simulink model "Encoder_Zynq"  (R2018a)
settings: Solver=ode3  StartTime=0.0  StopTime=SimulationsDauer  RelTol=1e-3  EnableMultiTasking=on
values from neighbouring files (symbols this model uses):
  f_ISR = 10000    [Script_Encoder_Zynq.m]
  IncPerTurn = 5000    [Script_Encoder_Zynq.m]
  n_max = 6000    [Script_Encoder_Zynq.m]
  OverSamplingFactor = 6    [Script_Encoder_Zynq.m]
  OverSamplingFactorInverse = 1/OverSamplingFactor    (= 0.166666666667)    [Script_Encoder_Zynq.m]
  Periode = 1/Striche_pro_Sekunde    (= 2.4e-06)    [Script_Encoder_Zynq.m]
  Phase_Delay_A = Periode/8    (= 3e-07)    [Script_Encoder_Zynq.m]
  Phase_Delay_B = -Periode/8    (= -3e-07)    [Script_Encoder_Zynq.m]
  PolePair = 4    [Script_Encoder_Zynq.m]
  T_mech = 2e-08    [Script_Encoder_Zynq.m]
  TestDrehzahl_rpm = 5000    [Script_Encoder_Zynq.m]
undefined symbols (not defined in the file or in its folder): DiscIntNeverNeededParam
libraries: dspswit3 x2, powerlib_meascontrol x2, simulink_extras x1, powerlib x1
(part 1 of 2)
settings Model: Creator=Wendel_ELSYS  LastModifiedBy=Wendel
settings DataIOCC: LimitDataPoints=on  SaveFormat=Array
settings OptimizationCC: BlockReduction=off  ConditionallyExecuteInputs=off  DefaultParameterBehavior=Inlined  LifeSpan=inf
settings DebuggingCC: AlgebraicLoopMsg=error  ParameterOverflowMsg=none  SFUnexpectedBacktrackingDiag=warning  SFNoUnconditionalDefaultTransitionDiag=warning  SFExecutionAtInitializationDiag=none
settings HardwareCC: ProdBitPerPointer=32  ProdBitPerSizeT=32  ProdBitPerPtrDiffT=32  ProdLargestAtomicFloat=None  ProdIntDivRoundTo=Undefined  ProdEndianess=Unspecified  ProdWordSize=32  ProdHWDeviceType=ASIC/FPGA->ASIC/FPGA  ProdEqTarget=off
settings ModelReferenceCC: PropagateSignalLabelsOutOfModel=off
settings CodeAppCC: StateflowObjectComments=on
settings GRTTargetCC: TargetLangStandard=C89/C90 (ANSI)  GeneratePreprocessorConditionals=Disable all
settings ConfigComp: CovMetricSettings=dw  CovHtmlReporting=on  CovSaveCumulativeToWorkspaceVar=on  CovSaveSingleToWorkspaceVar=on  CovExternalEMLEnable=off
settings SimscapeCC: SimscapeNormalizeSystem=off

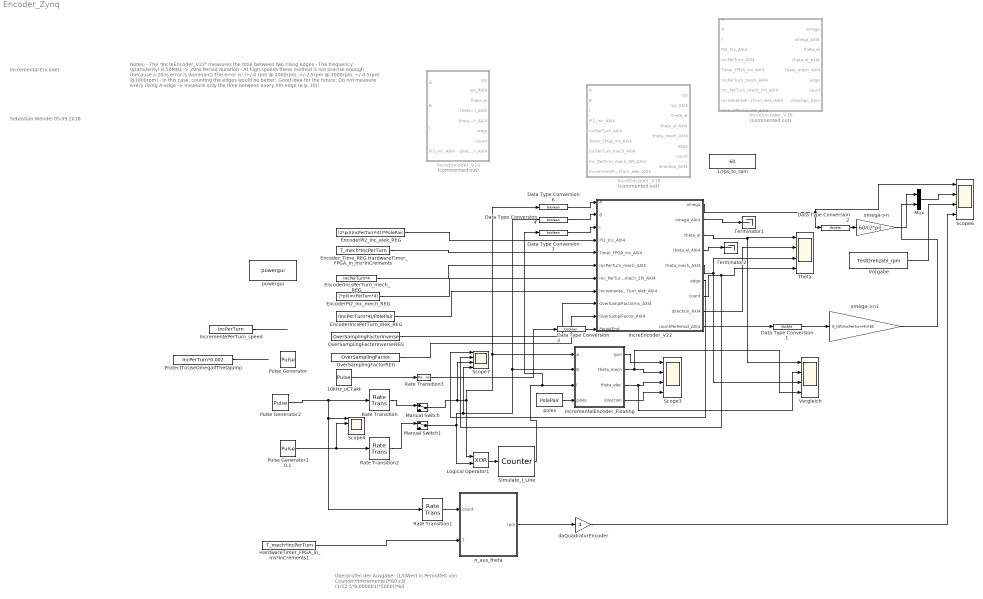
== system Encoder_Zynq ==
  note: Überprüfen der Ausgabe:
      | (1/((Wert in Periodfelt von Counter)*Inkremente))*60
      | z.B. (1/((2.5*0.000001)*5000))*60
  note: Sebastian Wendel
      | 05.09.2018
  note: Notes:
      | - The "IncreEncoder_V22" measures the time between two rising edges
      | - The frequency (granularity) is 50MHz -> 20ns Period duration
      | - At high speeds these method is not precise enough (because a 20ns error is dominant)
      | The error is: (+/-6 rpm @ 5000rpm, +/-2,5rpm @ 3000rpm, +/-0,5rpm @1000rpm)
      | - In this case, counting the edges would be better!
      |
      | Good idea for the future: Do not measure every rising A-edge
      | -> measure only the time between every Xth edge (e.g. 10)!
  note: Incremental Encoder
  1/rps_to_rpm : Constant  Value=60  OutDataTypeStr=double  SampleTime=T_mech
  10kHz_uCTakt : DiscretePulseGenerator  PulseType=Time based  Period=0.000100  PulseWidth=0.0002  SampleTime=T_mech  VectorParams1D=off
  Data Type Conversion1 : DataTypeConversion  OutDataTypeStr=double
  Data Type Conversion2 : DataTypeConversion  OutDataTypeStr=double
  Data Type Conversion{3..4,6..7} (4 alike) : DataTypeConversion  OutDataTypeStr=boolean
  "EncoderIncsPerTurn_elek_REG " : Constant  Value=(IncPerTurn*4)/PolePair  OutDataTypeStr=fixdt(0,16,0)  SampleTime=T_mech
  EncoderIncsPerTurn_mech_REG : Constant  Value=IncPerTurn*4  OutDataTypeStr=fixdt(0,16,0)  SampleTime=T_mech
  EncoderPI2_Inc_elek_REG : Constant  Value=(2*pi/(IncPerTurn*4))*PolePair  OutDataTypeStr=fixdt(0,24,24)  SampleTime=T_mech
  EncoderPI2_Inc_mech_REG : Constant  Value=2*pi/(IncPerTurn*4)  OutDataTypeStr=fixdt(0,24,24)  SampleTime=T_mech
  Encoder_Time_REG HardwareTimer_FPGA_in_ms*InCrements : Constant  Value=T_mech*IncPerTurn  OutDataTypeStr=fixdt(0,32,26)  SampleTime=T_mech
  HardwareTimer_FPGA_in_ms*InCrements1 : Constant  Value=T_mech*IncPerTurn  OutDataTypeStr=double  SampleTime=T_mech
  IncreEncoder_V16 : Subsystem  Commented=on  TreatAsAtomicUnit=on
  IncreEncoder_V18 : Subsystem  Commented=on  TreatAsAtomicUnit=on
  IncreEncoder_V19 : Subsystem  Commented=on  TreatAsAtomicUnit=on
  IncreEncoder_V22 : Subsystem  TreatAsAtomicUnit=on
  IncrementalEncoder_Floating : Subsystem
  IncrementePerTurn_speed : Constant  Value=IncPerTurn  OutDataTypeStr=fixdt(0,16,0)  SampleTime=T_mech
  Logical Operator1 : Logic  Operator=XOR  AllPortsSameDT=off  OutDataTypeStr=boolean
  Manual Switch : ManualSwitch
  Manual Switch1 : ManualSwitch
  Mux : Mux  Inputs=2
  OverSamplingFactorInverseREG : Constant  Value=OverSamplingFactorInverse  OutDataTypeStr=fixdt(0,16,15)  SampleTime=T_mech
  OverSamplingFactorREG : Constant  Value=OverSamplingFactor  OutDataTypeStr=fixdt(0,16,0)  SampleTime=T_mech
  ProtectToUseOmegaIfThetaJump : Constant  Value=IncPerTurn*0.002  OutDataTypeStr=uint16  SampleTime=T_mech
  Pulse Generator : DiscretePulseGenerator  PulseType=Time based  Period=0.01  PulseWidth=50  PhaseDelay=0.00000125  SampleTime=T_mech  VectorParams1D=off
  Pulse Generator1 0.1 : DiscretePulseGenerator  PulseType=Time based  Period=Periode  PulseWidth=50  PhaseDelay=Phase_Delay_B  SampleTime=T_mech  VectorParams1D=off
  Pulse Generator2 : DiscretePulseGenerator  PulseType=Time based  Period=Periode  PulseWidth=50  PhaseDelay=Phase_Delay_A  SampleTime=T_mech  VectorParams1D=off
  Rate Transition{,1..3} (4 alike) : RateTransition  Deterministic=off  OutPortSampleTime=T_mech
  Scope{3..4,6..7} (4 alike) : Scope  NumInputPorts=4
  Simulate_I_Line : dspswit3/Counter  Direction=Up  CountEvent=Either edge  CounterSize=User defined  MaxCount=IncPerTurn*4  InitialCount=0  Output=Hit  HitValue=IncPerTurn*4  ResetInput=off  SamplesPerFrame=1  Ts=1  CntDtype=double  HitDtype=Boolean
  Terminator1 : Terminator
  Terminator2 : Terminator
  Theta : Scope  NumInputPorts=4
  Vergleich : Scope  NumInputPorts=4
  Vorgabe : Constant  Value=TestDrehzahl_rpm
  "daQuadraturEncoder " : Gain  Gain=4
  n_aus_theta : Subsystem  TreatAsAtomicUnit=on
  omega->n : Gain  Gain=60/(2*pi)  OutDataTypeStr=double
  omega->n1 : Gain  Gain=(f_ISR/(IncPerTurn*4))*60  OutDataTypeStr=double
  poles : Constant  Value=PolePair  OutDataTypeStr=uint8  SampleTime=-1
  powergui : powerlib/powergui  Priority=1  SimulationMode=Discrete  SampleTime=T_mech  frequency=60  Iterations=50  frequencyindice=0  Pbase=100e6  ErrMax=1e-4  UnitsV=kV  UnitsW=MW  buscounter=0  FunctionMessages=off  echomessages=off  EnableUseOfTLC=off  CurrentSourceSwitches=off  DisableSnubberDevices=off  DisableRonSwitches=off  DisableVfSwitches=off  DisplayEquations=off  SolverType=Tustin  Interpol=off  ExternalGateDelay=off  methode=off  Ts=0  x0status=blocks  SPID=off  SwTol=0  HookPort=off  RestoreLinks=warning  ResistiveCurrentMeasurement=off  Frange=[0:2:500]  Ylog=off  Xlog=on  ShowGrid=off  save=off  variable=ZData  structure=0  ZoomFFT=on  StartTime=0.0  cycles=1  DisplayStyle=1  fundamental=60  FreqAxis=off  MaxFrequency=1000  frequencyindicesteady=1  RmsSteady=1  display=off
  wires:
  Pulse Generator1 0.1/1 -> Scope4/2, Rate Transition2/1
  Manual Switch1/1 -> Logical Operator1/2, Scope7/4, IncrementalEncoder_Floating/2(B), Data Type Conversion4/1
  Simulate_I_Line/1 -> IncrementalEncoder_Floating/3(I), Data Type Conversion7/1
  Logical Operator1/1 -> Simulate_I_Line/1
  Manual Switch/1 -> Scope7/3, Data Type Conversion6/1, IncrementalEncoder_Floating/1(A), Logical Operator1/1
  Data Type Conversion6/1 -> IncreEncoder_V22/1(A)
  Data Type Conversion4/1 -> IncreEncoder_V22/2(B)
  Data Type Conversion7/1 -> IncreEncoder_V22/3(I)
  IncreEncoder_V22/1(omega) -> Scope6/1, Data Type Conversion2/1
  IncreEncoder_V22/8(direction_AXI4) -> Theta/2
  IncreEncoder_V22/6(edge) -> Scope7/1
  IncreEncoder_V22/7(count) -> Theta/4, Scope7/2
  IncrementalEncoder_Floating/1(rpm) -> Scope3/1
  IncrementalEncoder_Floating/2(theta_mech) -> Vergleich/4, Scope3/2
  IncrementalEncoder_Floating/3(theta_elec) -> Vergleich/2, Scope3/3
  IncrementalEncoder_Floating/4(direction) -> Scope3/4
  poles/1 -> IncrementalEncoder_Floating/4(poles)
  EncoderPI2_Inc_elek_REG/1 -> IncreEncoder_V22/4(PI2_Inc_AXI4)
  IncreEncoder_V22/3(theta_el) -> Theta/1, Vergleich/1
  IncreEncoder_V22/5(theta_mech_AXI4) -> Vergleich/3, Theta/3
  IncreEncoder_V22/4(theta_el_AXI4) -> Terminator2/1
  IncreEncoder_V22/2(omega_AXI4) -> Terminator1/1
  Encoder_Time_REG HardwareTimer_FPGA_in_ms*InCrements/1 -> IncreEncoder_V22/5(Timer_FPGA_ms_AXI4)
  EncoderIncsPerTurn_mech_REG/1 -> IncreEncoder_V22/6(IncPerTurn_mech_AXI4)
  EncoderPI2_Inc_mech_REG/1 -> IncreEncoder_V22/7(Inc_PerTurn_mech_2PI_AXI4)
  IncrementePerTurn_speed/1 -> ?
  "EncoderIncsPerTurn_elek_REG "/1 -> IncreEncoder_V22/8(IncrementePerTurn_elek_AXI4)
  omega->n/1 -> Mux/1
  Data Type Conversion2/1 -> omega->n/1
  HardwareTimer_FPGA_in_ms*InCrements1/1 -> n_aus_theta/2(T)
  Rate Transition1/1 -> n_aus_theta/1(count)
  n_aus_theta/1(rpm) -> "daQuadraturEncoder "/1
  Pulse Generator2/1 -> Rate Transition/1, Scope4/1, Rate Transition1/1
  "daQuadraturEncoder "/1 -> Scope6/4
  ProtectToUseOmegaIfThetaJump/1 -> ?
  Vorgabe/1 -> Scope6/3
  OverSamplingFactorInverseREG/1 -> IncreEncoder_V22/9(OverSamplFactorInv_AXI4)
  OverSamplingFactorREG/1 -> IncreEncoder_V22/10(OverSamplFactor_AXI4)
  Rate Transition2/1 -> Manual Switch1/1
  Rate Transition/1 -> Manual Switch/1
  10kHz_uCTakt/1 -> Rate Transition3/1
  Rate Transition3/1 -> Data Type Conversion3/1
  Data Type Conversion1/1 -> omega->n1/1
  IncreEncoder_V22/9(countPerPeriod_AXI4) -> Data Type Conversion1/1
  Mux/1 -> Scope6/2
  omega->n1/1 -> Mux/2
  Data Type Conversion3/1 -> IncreEncoder_V22/11(PeriodEnd)

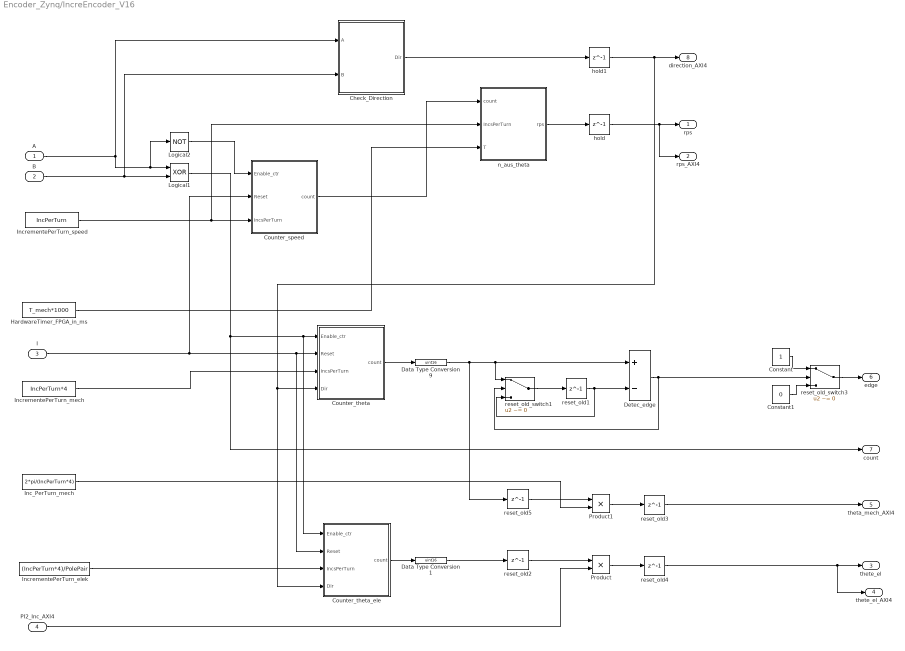
== system Encoder_Zynq/IncreEncoder_V16 ==
  A : Inport
  B : Inport  Port=2
  I : Inport  Port=3
  PI2_Inc_AXI4 : Inport  Port=4
  Check_Direction : Subsystem  TreatAsAtomicUnit=on
  Constant : Constant  OutDataTypeStr=boolean  SampleTime=-1
  Constant1 : Constant  Value=0  OutDataTypeStr=boolean  SampleTime=-1
  Counter_speed : Subsystem  TreatAsAtomicUnit=on
  Counter_theta : Subsystem  TreatAsAtomicUnit=on
  Counter_theta_ele : Subsystem  TreatAsAtomicUnit=on
  Data Type Conversion1 : DataTypeConversion  OutDataTypeStr=uint16
  Data Type Conversion9 : DataTypeConversion  OutDataTypeStr=uint16
  Detec_edge : Sum  Inputs=+-  AccumDataTypeStr=uint8  OutDataTypeStr=uint8
  HardwareTimer_FPGA_in_ms : Constant  Value=T_mech*1000  OutDataTypeStr=fixdt(0,30,24)  SampleTime=T_mech
  Inc_PerTurn_mech : Constant  Value=2*pi/(IncPerTurn*4)  OutDataTypeStr=fixdt(0,24,24)  SampleTime=T_mech
  IncrementePerTurn_elek : Constant  Value=(IncPerTurn*4)/PolePair  OutDataTypeStr=fixdt(0,16,0)  SampleTime=T_mech
  IncrementePerTurn_mech : Constant  Value=IncPerTurn*4  OutDataTypeStr=fixdt(0,16,0)  SampleTime=T_mech
  IncrementePerTurn_speed : Constant  Value=IncPerTurn  OutDataTypeStr=fixdt(0,16,0)  SampleTime=T_mech
  Logical1 : Logic  Operator=XOR  AllPortsSameDT=off  OutDataTypeStr=boolean
  Logical2 : Logic  Operator=NOT  AllPortsSameDT=off  OutDataTypeStr=boolean
  Product : Product  OutDataTypeStr=fixdt(0,24,20)
  Product1 : Product  OutDataTypeStr=fixdt(0,24,20)
  hold : Delay  DelayLength=1
  hold1 : Delay  DelayLength=1
  n_aus_theta : Subsystem  TreatAsAtomicUnit=on
  reset_old{1..5} (5 alike) : Delay  DelayLength=1
  reset_old_switch1 : Switch  Criteria=u2 ~= 0
  reset_old_switch3 : Switch  Criteria=u2 ~= 0
  rps : Outport
  rps_AXI4 : Outport  Port=2
  thete_el : Outport  Port=3
  thete_el_AXI4 : Outport  Port=4
  theta_mech_AXI4 : Outport  Port=5
  edge : Outport  Port=6
  count : Outport  Port=7
  direction_AXI4 : Outport  Port=8
  wires:
  A/1 -> Check_Direction/1(A), Logical2/1, Logical1/1
  B/1 -> Check_Direction/2(B), Logical1/2
  I/1 -> Counter_speed/2(Reset), Counter_theta_ele/2(Reset), Counter_theta/2(Reset)
  IncrementePerTurn_speed/1 -> Counter_speed/3(IncsPerTurn), n_aus_theta/2(IncsPerTurn)
  Check_Direction/1(Dir) -> hold1/1
  hold/1 -> rps_AXI4/1, rps/1
  hold1/1 -> Counter_theta_ele/4(Dir), Counter_theta/4(Dir), direction_AXI4/1
  Counter_theta/1(count) -> Data Type Conversion9/1
  reset_old_switch1/1 -> reset_old1/1
  reset_old1/1 -> reset_old_switch1/3, Detec_edge/2
  reset_old3/1 -> theta_mech_AXI4/1
  Product1/1 -> reset_old3/1
  Inc_PerTurn_mech/1 -> Product1/2
  Product/1 -> reset_old4/1
  Constant/1 -> reset_old_switch3/1
  reset_old_switch3/1 -> edge/1
  Constant1/1 -> reset_old_switch3/3
  Detec_edge/1 -> reset_old_switch3/2, reset_old_switch1/2
  Logical1/1 -> count/1, Counter_theta_ele/1(Enable_ctr), Counter_theta/1(Enable_ctr)
  Counter_speed/1(count) -> n_aus_theta/1(count)
  IncrementePerTurn_mech/1 -> Counter_theta/3(IncsPerTurn)
  n_aus_theta/1(rps) -> hold/1
  Data Type Conversion9/1 -> reset_old5/1, Detec_edge/1, reset_old_switch1/1
  IncrementePerTurn_elek/1 -> Counter_theta_ele/3(IncsPerTurn)
  PI2_Inc_AXI4/1 -> Product/2
  Counter_theta_ele/1(count) -> Data Type Conversion1/1
  reset_old4/1 -> thete_el_AXI4/1, thete_el/1
  Data Type Conversion1/1 -> reset_old2/1
  reset_old2/1 -> Product/1
  reset_old5/1 -> Product1/1
  Logical2/1 -> Counter_speed/1(Enable_ctr)
  HardwareTimer_FPGA_in_ms/1 -> n_aus_theta/3(T)

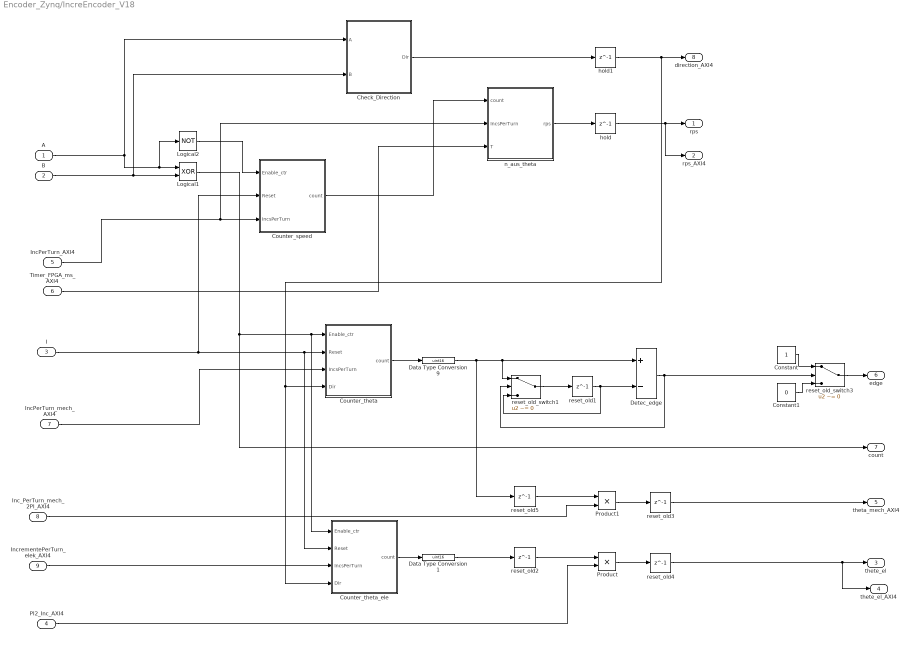
== system Encoder_Zynq/IncreEncoder_V18 ==
  A : Inport
  B : Inport  Port=2
  I : Inport  Port=3
  PI2_Inc_AXI4 : Inport  Port=4
  IncPerTurn_AXI4 : Inport  Port=5
  Timer_FPGA_ms_AXI4 : Inport  Port=6
  IncPerTurn_mech_AXI4 : Inport  Port=7
  Inc_PerTurn_mech_2PI_AXI4 : Inport  Port=8
  IncrementePerTurn_elek_AXI4 : Inport  Port=9
  Check_Direction : Subsystem  TreatAsAtomicUnit=on
  Constant : Constant  OutDataTypeStr=boolean  SampleTime=-1
  Constant1 : Constant  Value=0  OutDataTypeStr=boolean  SampleTime=-1
  Counter_speed : Subsystem  TreatAsAtomicUnit=on
  Counter_theta : Subsystem  TreatAsAtomicUnit=on
  Counter_theta_ele : Subsystem  TreatAsAtomicUnit=on
  Data Type Conversion1 : DataTypeConversion  OutDataTypeStr=uint16
  Data Type Conversion9 : DataTypeConversion  OutDataTypeStr=uint16
  Detec_edge : Sum  Inputs=+-  AccumDataTypeStr=uint8  OutDataTypeStr=uint8
  Logical1 : Logic  Operator=XOR  AllPortsSameDT=off  OutDataTypeStr=boolean
  Logical2 : Logic  Operator=NOT  AllPortsSameDT=off  OutDataTypeStr=boolean
  Product : Product  OutDataTypeStr=fixdt(1,24,20)
  Product1 : Product  OutDataTypeStr=fixdt(1,24,20)
  hold : Delay  DelayLength=1
  hold1 : Delay  DelayLength=1
  n_aus_theta : Subsystem  TreatAsAtomicUnit=on
  reset_old{1..5} (5 alike) : Delay  DelayLength=1
  reset_old_switch1 : Switch  Criteria=u2 ~= 0
  reset_old_switch3 : Switch  Criteria=u2 ~= 0
  rps : Outport
  rps_AXI4 : Outport  Port=2
  thete_el : Outport  Port=3
  thete_el_AXI4 : Outport  Port=4
  theta_mech_AXI4 : Outport  Port=5
  edge : Outport  Port=6
  count : Outport  Port=7
  direction_AXI4 : Outport  Port=8
  wires:
  A/1 -> Check_Direction/1(A), Logical2/1, Logical1/1
  B/1 -> Check_Direction/2(B), Logical1/2
  I/1 -> Counter_speed/2(Reset), Counter_theta_ele/2(Reset), Counter_theta/2(Reset)
  IncPerTurn_AXI4/1 -> Counter_speed/3(IncsPerTurn), n_aus_theta/2(IncsPerTurn)
  Check_Direction/1(Dir) -> hold1/1
  hold/1 -> rps_AXI4/1, rps/1
  hold1/1 -> Counter_theta_ele/4(Dir), Counter_theta/4(Dir), direction_AXI4/1
  Counter_theta/1(count) -> Data Type Conversion9/1
  reset_old_switch1/1 -> reset_old1/1
  reset_old1/1 -> reset_old_switch1/3, Detec_edge/2
  reset_old3/1 -> theta_mech_AXI4/1
  Product1/1 -> reset_old3/1
  Inc_PerTurn_mech_2PI_AXI4/1 -> Product1/2
  Product/1 -> reset_old4/1
  Constant/1 -> reset_old_switch3/1
  reset_old_switch3/1 -> edge/1
  Constant1/1 -> reset_old_switch3/3
  Detec_edge/1 -> reset_old_switch3/2, reset_old_switch1/2
  Logical1/1 -> count/1, Counter_theta_ele/1(Enable_ctr), Counter_theta/1(Enable_ctr)
  Counter_speed/1(count) -> n_aus_theta/1(count)
  IncPerTurn_mech_AXI4/1 -> Counter_theta/3(IncsPerTurn)
  n_aus_theta/1(rps) -> hold/1
  Data Type Conversion9/1 -> reset_old5/1, Detec_edge/1, reset_old_switch1/1
  IncrementePerTurn_elek_AXI4/1 -> Counter_theta_ele/3(IncsPerTurn)
  PI2_Inc_AXI4/1 -> Product/2
  Counter_theta_ele/1(count) -> Data Type Conversion1/1
  reset_old4/1 -> thete_el_AXI4/1, thete_el/1
  Data Type Conversion1/1 -> reset_old2/1
  reset_old2/1 -> Product/1
  reset_old5/1 -> Product1/1
  Logical2/1 -> Counter_speed/1(Enable_ctr)
  Timer_FPGA_ms_AXI4/1 -> n_aus_theta/3(T)

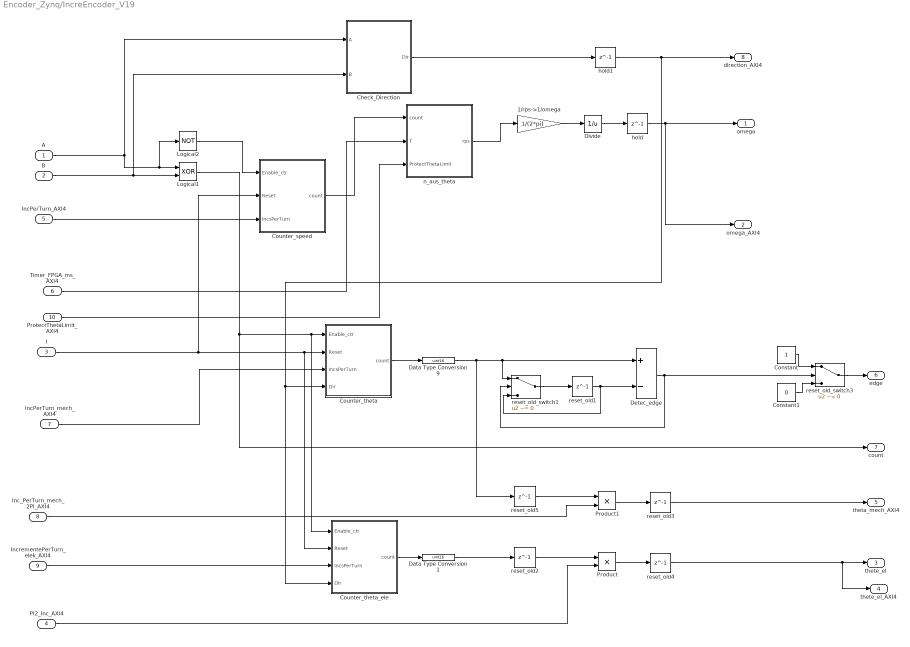
== system Encoder_Zynq/IncreEncoder_V19 ==
  A : Inport
  B : Inport  Port=2
  I : Inport  Port=3
  PI2_Inc_AXI4 : Inport  Port=4
  IncPerTurn_AXI4 : Inport  Port=5
  Timer_FPGA_ms_AXI4 : Inport  Port=6
  IncPerTurn_mech_AXI4 : Inport  Port=7
  Inc_PerTurn_mech_2PI_AXI4 : Inport  Port=8
  IncrementePerTurn_elek_AXI4 : Inport  Port=9
  ProtectThetaLimit_AXI4 : Inport  Port=10
  1/rps->1/omega : Gain  Gain=1/(2*pi)  OutDataTypeStr=fixdt(1,24,18)
  Check_Direction : Subsystem  TreatAsAtomicUnit=on
  Constant : Constant  OutDataTypeStr=boolean  SampleTime=-1
  Constant1 : Constant  Value=0  OutDataTypeStr=boolean  SampleTime=-1
  Counter_speed : Subsystem  TreatAsAtomicUnit=on
  Counter_theta : Subsystem  TreatAsAtomicUnit=on
  Counter_theta_ele : Subsystem  TreatAsAtomicUnit=on
  Data Type Conversion1 : DataTypeConversion  OutDataTypeStr=uint16
  Data Type Conversion9 : DataTypeConversion  OutDataTypeStr=uint16
  Detec_edge : Sum  Inputs=+-  AccumDataTypeStr=uint8  OutDataTypeStr=uint8
  Divide : Math  Operator=reciprocal  OutDataTypeStr=fixdt(1,24,11)  RndMeth=Zero  SaturateOnIntegerOverflow=on
  Logical1 : Logic  Operator=XOR  AllPortsSameDT=off  OutDataTypeStr=boolean
  Logical2 : Logic  Operator=NOT  AllPortsSameDT=off  OutDataTypeStr=boolean
  Product : Product  OutDataTypeStr=fixdt(1,24,20)
  Product1 : Product  OutDataTypeStr=fixdt(1,24,20)
  hold : Delay  DelayLength=1
  hold1 : Delay  DelayLength=1
  n_aus_theta : Subsystem  TreatAsAtomicUnit=on
  reset_old{1..5} (5 alike) : Delay  DelayLength=1
  reset_old_switch1 : Switch  Criteria=u2 ~= 0
  reset_old_switch3 : Switch  Criteria=u2 ~= 0
  omega : Outport
  omega_AXI4 : Outport  Port=2
  thete_el : Outport  Port=3
  thete_el_AXI4 : Outport  Port=4
  theta_mech_AXI4 : Outport  Port=5
  edge : Outport  Port=6
  count : Outport  Port=7
  direction_AXI4 : Outport  Port=8
  wires:
  A/1 -> Check_Direction/1(A), Logical2/1, Logical1/1
  B/1 -> Check_Direction/2(B), Logical1/2
  I/1 -> Counter_speed/2(Reset), Counter_theta_ele/2(Reset), Counter_theta/2(Reset)
  IncPerTurn_AXI4/1 -> Counter_speed/3(IncsPerTurn)
  Check_Direction/1(Dir) -> hold1/1
  hold/1 -> omega_AXI4/1, omega/1
  hold1/1 -> Counter_theta_ele/4(Dir), Counter_theta/4(Dir), direction_AXI4/1
  Counter_theta/1(count) -> Data Type Conversion9/1
  reset_old_switch1/1 -> reset_old1/1
  reset_old1/1 -> reset_old_switch1/3, Detec_edge/2
  reset_old3/1 -> theta_mech_AXI4/1
  Product1/1 -> reset_old3/1
  Inc_PerTurn_mech_2PI_AXI4/1 -> Product1/2
  Product/1 -> reset_old4/1
  Constant/1 -> reset_old_switch3/1
  reset_old_switch3/1 -> edge/1
  Constant1/1 -> reset_old_switch3/3
  Detec_edge/1 -> reset_old_switch3/2, reset_old_switch1/2
  Logical1/1 -> count/1, Counter_theta_ele/1(Enable_ctr), Counter_theta/1(Enable_ctr)
  Counter_speed/1(count) -> n_aus_theta/1(count)
  IncPerTurn_mech_AXI4/1 -> Counter_theta/3(IncsPerTurn)
  n_aus_theta/1(rps) -> 1/rps->1/omega/1
  Data Type Conversion9/1 -> reset_old5/1, Detec_edge/1, reset_old_switch1/1
  IncrementePerTurn_elek_AXI4/1 -> Counter_theta_ele/3(IncsPerTurn)
  PI2_Inc_AXI4/1 -> Product/2
  Counter_theta_ele/1(count) -> Data Type Conversion1/1
  reset_old4/1 -> thete_el_AXI4/1, thete_el/1
  Data Type Conversion1/1 -> reset_old2/1
  reset_old2/1 -> Product/1
  reset_old5/1 -> Product1/1
  Logical2/1 -> Counter_speed/1(Enable_ctr)
  Timer_FPGA_ms_AXI4/1 -> n_aus_theta/2(T)
  Divide/1 -> hold/1
  1/rps->1/omega/1 -> Divide/1
  ProtectThetaLimit_AXI4/1 -> n_aus_theta/3(ProtectThetaLimit)

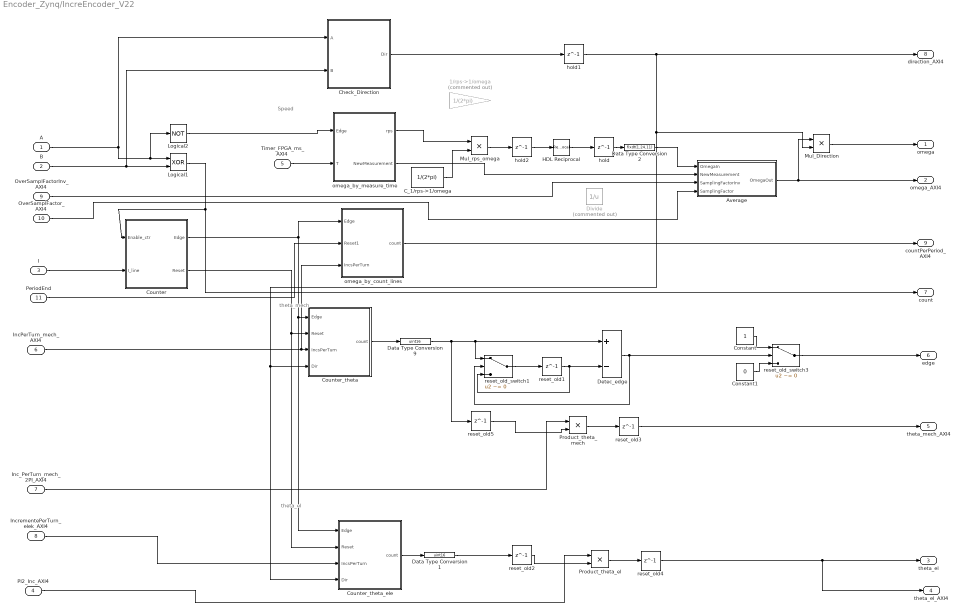
== system Encoder_Zynq/IncreEncoder_V22 ==
  note: Speed
  note: theta_mech
  note: theta_el
  A : Inport
  B : Inport  Port=2
  I : Inport  Port=3
  PI2_Inc_AXI4 : Inport  Port=4
  Timer_FPGA_ms_AXI4 : Inport  Port=5
  IncPerTurn_mech_AXI4 : Inport  Port=6
  Inc_PerTurn_mech_2PI_AXI4 : Inport  Port=7
  IncrementePerTurn_elek_AXI4 : Inport  Port=8
  OverSamplFactorInv_AXI4 : Inport  Port=9
  OverSamplFactor_AXI4 : Inport  Port=10
  PeriodEnd : Inport  Port=11
  1/rps->1/omega : Gain  Commented=on  Gain=1/(2*pi)  OutDataTypeStr=fixdt(1,24,18)
  Average : Subsystem
  C_1/rps->1/omega : Constant  Value=1/(2*pi)  OutDataTypeStr=fixdt(0,16,15)  SampleTime=-1
  Check_Direction : Subsystem  TreatAsAtomicUnit=on
  Constant : Constant  OutDataTypeStr=boolean  SampleTime=-1
  Constant1 : Constant  Value=0  OutDataTypeStr=boolean  SampleTime=-1
  Counter : Subsystem  TreatAsAtomicUnit=on
  Counter_theta : Subsystem  TreatAsAtomicUnit=on
  Counter_theta_ele : Subsystem  TreatAsAtomicUnit=on
  Data Type Conversion1 : DataTypeConversion  OutDataTypeStr=uint16
  Data Type Conversion2 : DataTypeConversion  OutDataTypeStr=fixdt(1,24,11)
  Data Type Conversion9 : DataTypeConversion  OutDataTypeStr=uint16
  Detec_edge : Sum  Inputs=+-  AccumDataTypeStr=uint8  OutDataTypeStr=uint8
  Divide : Math  Commented=on  Operator=reciprocal  OutDataTypeStr=fixdt(1,24,11)  RndMeth=Zero  SaturateOnIntegerOverflow=on
  HDL Reciprocal : Reciprocal
  Logical1 : Logic  Operator=XOR  AllPortsSameDT=off  OutDataTypeStr=boolean
  Logical2 : Logic  Operator=NOT  AllPortsSameDT=off  OutDataTypeStr=boolean
  Mul_Direction : Product  Inputs=**  SaturateOnIntegerOverflow=on  RndMeth=Zero  OutDataTypeStr=Inherit: Same as first input
  Mul_rps_omega : Product  Inputs=**  SaturateOnIntegerOverflow=on  RndMeth=Zero  OutDataTypeStr=Inherit: Same as first input
  Product_theta_el : Product  OutDataTypeStr=fixdt(1,24,20)
  Product_theta_mech : Product  OutDataTypeStr=fixdt(1,24,20)
  hold : Delay  DelayLength=1
  hold1 : Delay  DelayLength=1
  hold2 : Delay  DelayLength=1
  omega_by_count_lines : Subsystem  TreatAsAtomicUnit=on
  omega_by_measure_time : Subsystem  TreatAsAtomicUnit=on
  reset_old{1..5} (5 alike) : Delay  DelayLength=1
  reset_old_switch1 : Switch  Criteria=u2 ~= 0
  reset_old_switch3 : Switch  Criteria=u2 ~= 0
  omega : Outport
  omega_AXI4 : Outport  Port=2
  theta_el : Outport  Port=3
  theta_el_AXI4 : Outport  Port=4
  theta_mech_AXI4 : Outport  Port=5
  edge : Outport  Port=6
  count : Outport  Port=7
  direction_AXI4 : Outport  Port=8
  countPerPeriod_AXI4 : Outport  Port=9
  wires:
  A/1 -> Check_Direction/1(A), Logical2/1, Logical1/1
  B/1 -> Check_Direction/2(B), Logical1/2
  I/1 -> Counter/2(I_line)
  hold/1 -> Data Type Conversion2/1
  hold1/1 -> Mul_Direction/2, Counter_theta_ele/4(Dir), Counter_theta/4(Dir), direction_AXI4/1
  Counter_theta/1(count) -> Data Type Conversion9/1
  reset_old_switch1/1 -> reset_old1/1
  reset_old1/1 -> reset_old_switch1/3, Detec_edge/2
  reset_old3/1 -> theta_mech_AXI4/1
  Product_theta_mech/1 -> reset_old3/1
  Inc_PerTurn_mech_2PI_AXI4/1 -> Product_theta_mech/1
  Product_theta_el/1 -> reset_old4/1
  Constant/1 -> reset_old_switch3/1
  reset_old_switch3/1 -> edge/1
  Constant1/1 -> reset_old_switch3/3
  Detec_edge/1 -> reset_old_switch3/2, reset_old_switch1/2
  Logical1/1 -> count/1, Counter/1(Enable_ctr)
  IncPerTurn_mech_AXI4/1 -> omega_by_count_lines/3(IncsPerTurn), Counter_theta/3(IncsPerTurn)
  omega_by_measure_time/1(rps) -> Mul_rps_omega/1
  Data Type Conversion9/1 -> reset_old5/1, Detec_edge/1, reset_old_switch1/1
  IncrementePerTurn_elek_AXI4/1 -> Counter_theta_ele/3(IncsPerTurn)
  PI2_Inc_AXI4/1 -> Product_theta_el/1
  Counter_theta_ele/1(count) -> Data Type Conversion1/1
  reset_old4/1 -> theta_el_AXI4/1, theta_el/1
  Data Type Conversion1/1 -> reset_old2/1
  reset_old2/1 -> Product_theta_el/2
  reset_old5/1 -> Product_theta_mech/2
  Logical2/1 -> omega_by_measure_time/1(Edge)
  Timer_FPGA_ms_AXI4/1 -> omega_by_measure_time/2(T)
  HDL Reciprocal/1 -> hold/1
  Mul_rps_omega/1 -> hold2/1
  Mul_Direction/1 -> omega/1
  Counter/2(Reset) -> Counter_theta_ele/2(Reset), Counter_theta/2(Reset)
  Counter/1(Edge) -> omega_by_count_lines/1(Edge), Counter_theta_ele/1(Edge), Counter_theta/1(Edge)
  C_1/rps->1/omega/1 -> Mul_rps_omega/2
  hold2/1 -> HDL Reciprocal/1
  Check_Direction/1(Dir) -> hold1/1
  OverSamplFactorInv_AXI4/1 -> Average/3(SamplingFactorInv)
  omega_by_measure_time/2(NewMeasurement) -> Average/2(NewMeasurement)
  OverSamplFactor_AXI4/1 -> Average/4(SamplingFactor)
  Average/1(OmegaOut) -> omega_AXI4/1, Mul_Direction/1
  Data Type Conversion2/1 -> Average/1("OmegaIn ")
  PeriodEnd/1 -> omega_by_count_lines/2(Reset1)
  omega_by_count_lines/1(count) -> countPerPeriod_AXI4/1

== system Encoder_Zynq/IncrementalEncoder_Floating ==
  A : Inport
  B : Inport  Port=2
  I : Inport  Port=3
  poles : Inport  Port=4
  Add : Sum  Inputs=+-  OutDataTypeStr=fixdt(1,16,0)
  Counter3 : dspswit3/Counter  Direction=Up  CountEvent=Either edge  CounterSize=User defined  MaxCount=IncPerTurn*4  InitialCount=0  Output=Count  HitValue=32  ResetInput=on  SamplesPerFrame=1  Ts=1  CntDtype=double  HitDtype=Logical
  CutTheta_0_2PI : Subsystem
  Edge Detector2 : powerlib_meascontrol/Logic/Edge Detector  model=Rising  ic=0  Ts=-1
      settings: SourceProductName=Simscape Power Systems  SourceProductBaseCode=PS
  Edge Detector3 : powerlib_meascontrol/Logic/Edge Detector  model=Rising  ic=0  Ts=-1
      settings: SourceProductName=Simscape Power Systems  SourceProductBaseCode=PS
  Logical Operator1 : Logic  Operator=XOR  AllPortsSameDT=off  OutDataTypeStr=boolean
  Logical Operator3 : Logic  AllPortsSameDT=off  OutDataTypeStr=boolean
  Logical Operator4 : Logic  Operator=NOT  AllPortsSameDT=off  OutDataTypeStr=boolean
  Logical Operator5 : Logic  AllPortsSameDT=off  OutDataTypeStr=boolean
  Logical Operator6 : Logic  Operator=NOT  AllPortsSameDT=off  OutDataTypeStr=boolean
  Product : Product
  S-R Flip-Flop1 : simulink_extras/Flip Flops/S-R Flip-Flop  initial_condition=0
  Scope1 : Scope  NumInputPorts=4
  cut_theta_2pi : Gain  Gain=(2*pi)/IncPerTurn
  cut_theta_2pi1 : Gain  Gain=(2*pi)/IncPerTurn
  n_aus_theta_v4 : Subsystem
  rpm : Outport
  theta_mech : Outport  Port=2
  theta_elec : Outport  Port=3
  direction : Outport  Port=4
  wires:
  I/1 -> Counter3/2
  Counter3/1 -> cut_theta_2pi/1, Product/1, Scope1/1
  n_aus_theta_v4/1(n) -> rpm/1
  Logical Operator1/1 -> Scope1/4, Counter3/1
  cut_theta_2pi/1 -> Scope1/2, n_aus_theta_v4/1(theta), theta_mech/1
  Product/1 -> cut_theta_2pi1/1
  poles/1 -> Product/2
  cut_theta_2pi1/1 -> CutTheta_0_2PI/1(In1)
  CutTheta_0_2PI/1(Out1) -> theta_elec/1
  Edge Detector2/1 -> Logical Operator3/1
  Logical Operator4/1 -> Logical Operator3/2
  Logical Operator3/1 -> S-R Flip-Flop1/1
  Edge Detector3/1 -> Logical Operator5/1
  Logical Operator6/1 -> Logical Operator5/2
  Logical Operator5/1 -> S-R Flip-Flop1/2
  S-R Flip-Flop1/1 -> Add/1
  S-R Flip-Flop1/2 -> Add/2
  A/1 -> Logical Operator6/1, Edge Detector2/1, Logical Operator1/1
  B/1 -> Edge Detector3/1, Logical Operator4/1, Logical Operator1/2
  Add/1 -> direction/1

== system Encoder_Zynq/n_aus_theta ==
  count : Inport
  T : Inport  Port=2
  1/rps->1/omega : Gain  Gain=1/(2*pi)  OutDataTypeStr=double
  Add : Sum  Inputs=+-
  Add1 : Sum
  Constant : Constant  Value=0  OutDataTypeStr=double  SampleTime=-1
  Constant1 : Constant  Value=0  OutDataTypeStr=double  SampleTime=-1
  Constant2 : Constant  Value=0  OutDataTypeStr=double  SampleTime=-1
  Divide1 : Product  Inputs=/
  ProtectOverflow_T_count : Switch  Threshold=50
  ProtectOverflow_rps : Switch  Threshold=50  OutDataTypeStr=double
  Scope1 : Scope  NumInputPorts=4
  Scope2 : Scope  NumInputPorts=4
  T_count : Delay  DelayLength=1
  T_count_switch : Switch  Criteria=u2 ~= 0
  count_old : Delay  DelayLength=1
  count_old_switch : Switch  Criteria=u2 ~= 0
  speed_old : Delay  DelayLength=1
  speed_old_switch : Switch  Criteria=u2 ~= 0
  rpm : Outport
  wires:
  count_old_switch/1 -> count_old/1
  count_old/1 -> count_old_switch/3, Add/2
  Constant/1 -> T_count_switch/1
  Add/1 -> speed_old_switch/2, count_old_switch/2, Scope1/1, T_count_switch/2
  Constant1/1 -> ProtectOverflow_T_count/1
  ProtectOverflow_rps/1 -> 1/rps->1/omega/1, Scope2/1
  Constant2/1 -> ProtectOverflow_rps/1
  speed_old_switch/1 -> ProtectOverflow_rps/3, Scope2/3, speed_old/1
  speed_old/1 -> speed_old_switch/3
  T/1 -> Scope2/4, Add1/1
  ProtectOverflow_T_count/1 -> T_count/1
  T_count/1 -> Scope1/4, Add1/2
  Add1/1 -> Scope2/2, speed_old_switch/1, T_count_switch/3
  count/1 -> Add/1, count_old_switch/1
  T_count_switch/1 -> ProtectOverflow_rps/2, Scope1/2, ProtectOverflow_T_count/2, ProtectOverflow_T_count/3
  1/rps->1/omega/1 -> Divide1/1
  Divide1/1 -> rpm/1

== system Encoder_Zynq/IncreEncoder_V16/Check_Direction ==
  A : Inport
  B : Inport  Port=2
  Add : Sum  Inputs=+-  AccumDataTypeStr=fixdt(1,4,0)  OutDataTypeStr=fixdt(1,4,0)
  Add1 : Sum  Inputs=+-  AccumDataTypeStr=fixdt(1,4,0)  OutDataTypeStr=fixdt(1,4,0)
  Add2 : Sum  AccumDataTypeStr=fixdt(1,4,0)  OutDataTypeStr=fixdt(1,4,0)
  Change : Sum  AccumDataTypeStr=fixdt(1,4,0)  OutDataTypeStr=fixdt(1,4,0)
  Change1 : Delay  DelayLength=1
  Save_Direction : Switch  Criteria=u2 ~= 0  Threshold=0.1  OutDataTypeStr=Inherit: Inherit via back propagation
  Scope6 : Scope  NumInputPorts=4
  T_count_switch : Switch  Threshold=1  OutDataTypeStr=Inherit: Inherit via back propagation
  TrnLeft : Sum  Inputs=+-  AccumDataTypeStr=fixdt(1,4,0)  OutDataTypeStr=fixdt(1,4,0)
  TrnRight : Sum  Inputs=+-  AccumDataTypeStr=fixdt(1,4,0)  OutDataTypeStr=fixdt(1,4,0)
  TurnLeft : Constant  Value=-1  OutDataTypeStr=fixdt(1,4,0)  SampleTime=-1
  TurnRight : Constant  OutDataTypeStr=fixdt(1,4,0)  SampleTime=-1
  count_old : Delay  DelayLength=1
  count_old1 : Delay  DelayLength=1
  count_old2 : Delay  DelayLength=1
  count_old_switch : Switch  Criteria=u2 ~= 0  OutDataTypeStr=Inherit: Inherit via back propagation
  count_old_switch1 : Switch  Criteria=u2 ~= 0  OutDataTypeStr=Inherit: Inherit via back propagation
  new_value : Delay  DelayLength=1
  nothing : Constant  Value=0  OutDataTypeStr=fixdt(1,4,0)  SampleTime=-1
  nothing1 : Constant  Value=0  OutDataTypeStr=fixdt(1,4,0)  SampleTime=-1
  speed_old_switch : Switch  Threshold=1  OutDataTypeStr=Inherit: Inherit via back propagation
  Dir : Outport
  wires:
  A/1 -> TrnLeft/2, Add/1, count_old_switch/1
  count_old_switch/1 -> count_old/1
  count_old/1 -> count_old_switch/3, Add/2
  TurnRight/1 -> T_count_switch/1
  Add/1 -> TrnRight/1, count_old_switch/2
  T_count_switch/1 -> Change/1, Add2/1
  Save_Direction/1 -> count_old2/1
  B/1 -> TrnRight/2, Add1/1, count_old_switch1/1
  count_old_switch1/1 -> count_old1/1
  count_old1/1 -> count_old_switch1/3, Add1/2
  Add1/1 -> TrnLeft/1, count_old_switch1/2
  TrnRight/1 -> Scope6/1, T_count_switch/2
  new_value/1 -> Save_Direction/1
  TrnLeft/1 -> speed_old_switch/2, Scope6/2
  TurnLeft/1 -> speed_old_switch/1
  nothing/1 -> speed_old_switch/3
  nothing1/1 -> T_count_switch/3
  speed_old_switch/1 -> Change/2, Add2/2
  Add2/1 -> Scope6/4, new_value/1
  Change/1 -> Change1/1
  Change1/1 -> Scope6/3, Save_Direction/2
  count_old2/1 -> Save_Direction/3, Dir/1

== system Encoder_Zynq/IncreEncoder_V16/Counter_speed ==
  note: 1 for one cycle if edge recognized
  note: Check if count is to small
  note: Check if count is to big
  note: Reset
  note: Count
  Enable_ctr : Inport
  Reset : Inport  Port=2
  IncsPerTurn : Inport  Port=3
  Add1 : Sum  AccumDataTypeStr=int16  OutDataTypeStr=uint16
  Constant1 : Constant  Value=0  OutDataTypeStr=uint16  SampleTime=-1
  Constant2 : Constant  OutDataTypeStr=int8  SampleTime=-1
  Constant3 : Constant  Value=0  OutDataTypeStr=int8  SampleTime=-1
  Constant4 : Constant  Value=10  OutDataTypeStr=uint16  SampleTime=-1
  Detec_edge : Sum  Inputs=+-  AccumDataTypeStr=int8  OutDataTypeStr=int8
  Relational Operator : RelationalOperator  OutDataTypeStr=boolean  RndMeth=Nearest
  Reset_flag : Sum  Inputs=+-  AccumDataTypeStr=uint8  OutDataTypeStr=uint8
  Reset_when_overflow : Sum
  Resett_switch1 : Switch  Criteria=u2 ~= 0
  Resett_switch2 : Switch  Criteria=u2 ~= 0
  reset_old{,1..3} (4 alike) : Delay  DelayLength=1
  reset_old_switch : Switch  Criteria=u2 ~= 0
  reset_old_switch1 : Switch  Criteria=u2 ~= 0
  speed_old_switch1 : Switch  Threshold=1
  count : Outport
  wires:
  Reset/1 -> Reset_flag/1, reset_old_switch/1
  reset_old_switch/1 -> reset_old/1
  reset_old/1 -> reset_old_switch/3, Reset_flag/2
  Reset_flag/1 -> reset_old_switch/2, Resett_switch2/2
  Enable_ctr/1 -> Detec_edge/1, reset_old_switch1/1
  reset_old_switch1/1 -> reset_old1/1
  reset_old1/1 -> reset_old_switch1/3, Detec_edge/2
  Detec_edge/1 -> speed_old_switch1/2, reset_old_switch1/2  "1 for one cycle if edge recognized"
  Add1/1 -> Resett_switch2/3
  reset_old2/1 -> Relational Operator/1, Add1/2, count/1
  speed_old_switch1/1 -> Add1/1
  Constant3/1 -> speed_old_switch1/3
  Constant2/1 -> speed_old_switch1/1
  Constant4/1 -> Reset_when_overflow/1
  Reset_when_overflow/1 -> reset_old3/1
  Resett_switch1/1 -> reset_old2/1
  Relational Operator/1 -> Resett_switch1/2
  Constant1/1 -> Resett_switch2/1, Resett_switch1/1
  IncsPerTurn/1 -> Reset_when_overflow/2
  Resett_switch2/1 -> Resett_switch1/3
  reset_old3/1 -> Relational Operator/2

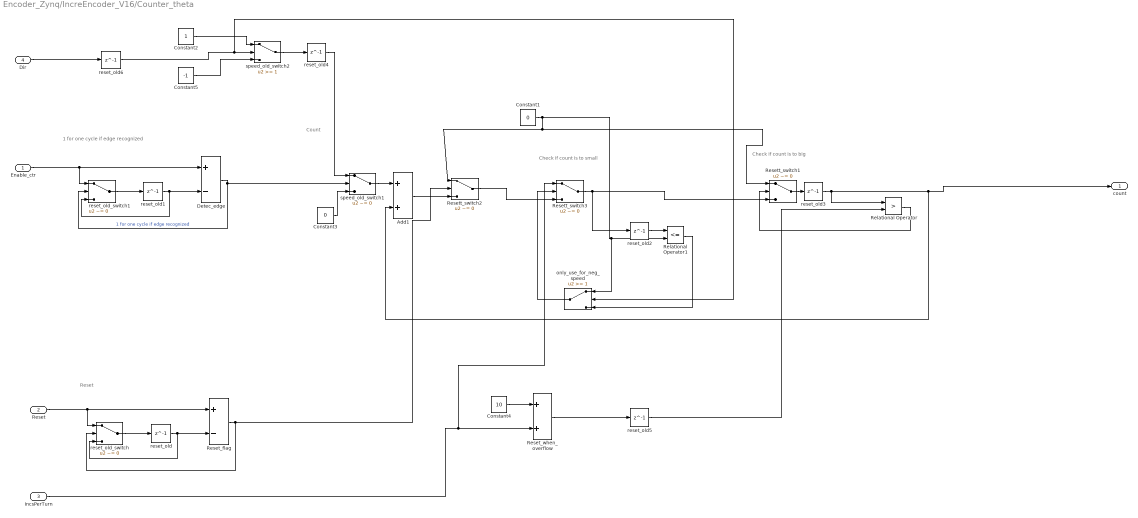
== system Encoder_Zynq/IncreEncoder_V16/Counter_theta ==
  note: 1 for one cycle if edge recognized
  note: Reset
  note: Count
  note: Check if count is to big
  note: Check if count is to small
  Enable_ctr : Inport
  Reset : Inport  Port=2
  IncsPerTurn : Inport  Port=3
  Dir : Inport  Port=4
  Add1 : Sum  AccumDataTypeStr=int16  OutDataTypeStr=int16
  Constant1 : Constant  Value=0  OutDataTypeStr=int16  SampleTime=-1
  Constant2 : Constant  OutDataTypeStr=int16  SampleTime=-1
  Constant3 : Constant  Value=0  OutDataTypeStr=int16  SampleTime=-1
  Constant4 : Constant  Value=10  OutDataTypeStr=int16  SampleTime=-1
  Constant5 : Constant  Value=-1  OutDataTypeStr=int16  SampleTime=-1
  Detec_edge : Sum  Inputs=+-  AccumDataTypeStr=int8  OutDataTypeStr=int8
  Relational Operator : RelationalOperator  Operator=>  OutDataTypeStr=boolean  RndMeth=Nearest
  Relational Operator1 : RelationalOperator  Operator=<=  OutDataTypeStr=boolean  RndMeth=Nearest
  Reset_flag : Sum  Inputs=+-  AccumDataTypeStr=uint8  OutDataTypeStr=uint8
  Reset_when_overflow : Sum  OutDataTypeStr=int16
  Resett_switch1 : Switch  Criteria=u2 ~= 0  OutDataTypeStr=int16
  Resett_switch2 : Switch  Criteria=u2 ~= 0  OutDataTypeStr=int16
  Resett_switch3 : Switch  Criteria=u2 ~= 0  OutDataTypeStr=int16
  only_use_for_neg_speed : Switch  Threshold=1
  reset_old{,1..6} (7 alike) : Delay  DelayLength=1
  reset_old_switch : Switch  Criteria=u2 ~= 0
  reset_old_switch1 : Switch  Criteria=u2 ~= 0
  speed_old_switch1 : Switch  Criteria=u2 ~= 0
  speed_old_switch2 : Switch  Threshold=1
  count : Outport
  wires:
  Reset/1 -> Reset_flag/1, reset_old_switch/1
  reset_old_switch/1 -> reset_old/1
  reset_old/1 -> reset_old_switch/3, Reset_flag/2
  Reset_flag/1 -> reset_old_switch/2, Resett_switch2/2
  Enable_ctr/1 -> Detec_edge/1, reset_old_switch1/1
  reset_old_switch1/1 -> reset_old1/1
  reset_old1/1 -> reset_old_switch1/3, Detec_edge/2
  Detec_edge/1 -> speed_old_switch1/2, reset_old_switch1/2  "1 for one cycle if edge recognized"
  Add1/1 -> Resett_switch2/3
  speed_old_switch1/1 -> Add1/1
  Constant3/1 -> speed_old_switch1/3
  Constant2/1 -> speed_old_switch2/1
  Constant4/1 -> Reset_when_overflow/1
  Reset_when_overflow/1 -> reset_old5/1
  IncsPerTurn/1 -> Resett_switch3/1, Reset_when_overflow/2
  Dir/1 -> reset_old6/1
  Constant5/1 -> speed_old_switch2/3
  speed_old_switch2/1 -> reset_old4/1
  reset_old3/1 -> Add1/2, count/1, Relational Operator/1
  Resett_switch1/1 -> reset_old3/1
  Relational Operator/1 -> Resett_switch1/2
  Constant1/1 -> Resett_switch2/1, Resett_switch1/1, only_use_for_neg_speed/1, Relational Operator1/2
  Resett_switch3/1 -> reset_old2/1, Resett_switch1/3
  Resett_switch2/1 -> Resett_switch3/3
  reset_old2/1 -> Relational Operator1/1
  Relational Operator1/1 -> only_use_for_neg_speed/3
  only_use_for_neg_speed/1 -> Resett_switch3/2
  reset_old4/1 -> speed_old_switch1/1
  reset_old5/1 -> Relational Operator/2
  reset_old6/1 -> only_use_for_neg_speed/2, speed_old_switch2/2

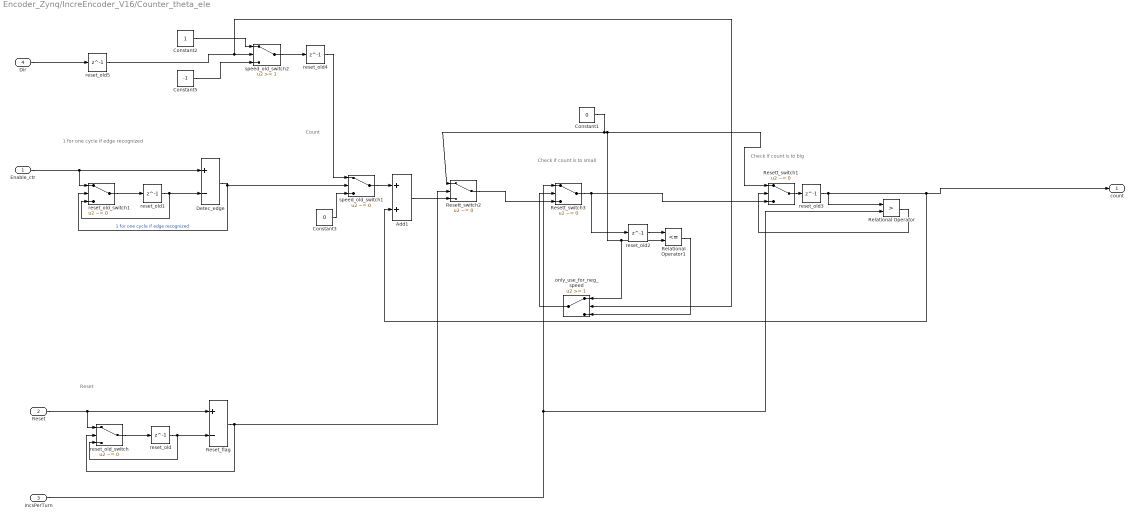
== system Encoder_Zynq/IncreEncoder_V16/Counter_theta_ele ==
  note: 1 for one cycle if edge recognized
  note: Reset
  note: Count
  note: Check if count is to big
  note: Check if count is to small
  Enable_ctr : Inport
  Reset : Inport  Port=2
  IncsPerTurn : Inport  Port=3
  Dir : Inport  Port=4
  Add1 : Sum  AccumDataTypeStr=int16  OutDataTypeStr=int16
  Constant1 : Constant  Value=0  OutDataTypeStr=int16  SampleTime=-1
  Constant2 : Constant  OutDataTypeStr=int16  SampleTime=-1
  Constant3 : Constant  Value=0  OutDataTypeStr=int16  SampleTime=-1
  Constant5 : Constant  Value=-1  OutDataTypeStr=int16  SampleTime=-1
  Detec_edge : Sum  Inputs=+-  AccumDataTypeStr=int8  OutDataTypeStr=int8
  Relational Operator : RelationalOperator  Operator=>  OutDataTypeStr=boolean  RndMeth=Nearest
  Relational Operator1 : RelationalOperator  Operator=<=  OutDataTypeStr=boolean  RndMeth=Nearest
  Reset_flag : Sum  Inputs=+-  AccumDataTypeStr=uint8  OutDataTypeStr=uint8
  Resett_switch1 : Switch  Criteria=u2 ~= 0  OutDataTypeStr=int16
  Resett_switch2 : Switch  Criteria=u2 ~= 0  OutDataTypeStr=int16
  Resett_switch3 : Switch  Criteria=u2 ~= 0  OutDataTypeStr=int16
  only_use_for_neg_speed : Switch  Threshold=1
  reset_old{,1..5} (6 alike) : Delay  DelayLength=1
  reset_old_switch : Switch  Criteria=u2 ~= 0
  reset_old_switch1 : Switch  Criteria=u2 ~= 0
  speed_old_switch1 : Switch  Criteria=u2 ~= 0
  speed_old_switch2 : Switch  Threshold=1
  count : Outport
  wires:
  Reset/1 -> Reset_flag/1, reset_old_switch/1
  reset_old_switch/1 -> reset_old/1
  reset_old/1 -> reset_old_switch/3, Reset_flag/2
  Reset_flag/1 -> reset_old_switch/2, Resett_switch2/2
  Enable_ctr/1 -> Detec_edge/1, reset_old_switch1/1
  reset_old_switch1/1 -> reset_old1/1
  reset_old1/1 -> reset_old_switch1/3, Detec_edge/2
  Detec_edge/1 -> speed_old_switch1/2, reset_old_switch1/2  "1 for one cycle if edge recognized"
  Add1/1 -> Resett_switch2/3
  speed_old_switch1/1 -> Add1/1
  Constant3/1 -> speed_old_switch1/3
  Constant2/1 -> speed_old_switch2/1
  IncsPerTurn/1 -> Resett_switch3/1, Relational Operator/2
  Dir/1 -> reset_old5/1
  Constant5/1 -> speed_old_switch2/3
  speed_old_switch2/1 -> reset_old4/1
  reset_old3/1 -> Add1/2, count/1, Relational Operator/1
  Resett_switch1/1 -> reset_old3/1
  Relational Operator/1 -> Resett_switch1/2
  Constant1/1 -> Resett_switch2/1, only_use_for_neg_speed/1, Relational Operator1/2, Resett_switch1/1
  Resett_switch3/1 -> reset_old2/1, Resett_switch1/3
  Resett_switch2/1 -> Resett_switch3/3
  reset_old2/1 -> Relational Operator1/1
  Relational Operator1/1 -> only_use_for_neg_speed/3
  only_use_for_neg_speed/1 -> Resett_switch3/2
  reset_old4/1 -> speed_old_switch1/1
  reset_old5/1 -> speed_old_switch2/2, only_use_for_neg_speed/2

== system Encoder_Zynq/IncreEncoder_V16/n_aus_theta ==
  count : Inport
  IncsPerTurn : Inport  Port=2
  T : Inport  Port=3
  Add : Sum  Inputs=+-
  Add1 : Sum
  Constant : Constant  Value=0  OutDataTypeStr=fixdt(0,30,24)  SampleTime=-1
  Constant1 : Constant  Value=0  OutDataTypeStr=fixdt(0,30,24)  SampleTime=-1
  Constant2 : Constant  Value=0  OutDataTypeStr=fixdt(0,30,24)  SampleTime=-1
  Gain : Gain  Gain=0.001  ParamDataTypeStr=fixdt(0,16)  OutMin=0  OutMax=0.001*2^16  OutDataTypeStr=fixdt(0,18)
  Product : Product  OutDataTypeStr=Inherit: Same as first input
  ProtectOverflow_T_count : Switch  Threshold=50
  ProtectOverflow_rps : Switch  Threshold=50  OutDataTypeStr=fixdt(0,30,24)
  T_count : Delay  DelayLength=1
  T_count_switch : Switch  Criteria=u2 ~= 0
  count_old : Delay  DelayLength=1
  count_old_switch : Switch  Criteria=u2 ~= 0
  speed_old : Delay  DelayLength=1
  speed_old_switch : Switch  Criteria=u2 ~= 0
  rps : Outport
  wires:
  count_old_switch/1 -> count_old/1
  count_old/1 -> count_old_switch/3, Add/2
  Constant/1 -> T_count_switch/1
  Add/1 -> speed_old_switch/2, count_old_switch/2, T_count_switch/2
  Constant1/1 -> ProtectOverflow_T_count/1
  ProtectOverflow_rps/1 -> rps/1
  Constant2/1 -> ProtectOverflow_rps/1
  speed_old_switch/1 -> ProtectOverflow_rps/3, speed_old/1
  speed_old/1 -> speed_old_switch/3
  IncsPerTurn/1 -> Gain/1
  Gain/1 -> Product/2
  T/1 -> Add1/1
  ProtectOverflow_T_count/1 -> T_count/1
  T_count/1 -> Add1/2
  Product/1 -> speed_old_switch/1
  Add1/1 -> Product/1, T_count_switch/3
  count/1 -> Add/1, count_old_switch/1
  T_count_switch/1 -> ProtectOverflow_rps/2, ProtectOverflow_T_count/2, ProtectOverflow_T_count/3

== system Encoder_Zynq/IncreEncoder_V18/Check_Direction ==
  A : Inport
  B : Inport  Port=2
  Add : Sum  Inputs=+-  AccumDataTypeStr=fixdt(1,4,0)  OutDataTypeStr=fixdt(1,4,0)
  Add1 : Sum  Inputs=+-  AccumDataTypeStr=fixdt(1,4,0)  OutDataTypeStr=fixdt(1,4,0)
  Add2 : Sum  AccumDataTypeStr=fixdt(1,4,0)  OutDataTypeStr=fixdt(1,4,0)
  Change : Sum  AccumDataTypeStr=fixdt(1,4,0)  OutDataTypeStr=fixdt(1,4,0)
  Change1 : Delay  DelayLength=1
  Save_Direction : Switch  Criteria=u2 ~= 0  Threshold=0.1  OutDataTypeStr=Inherit: Inherit via back propagation
  Scope6 : Scope  NumInputPorts=4
  T_count_switch : Switch  Threshold=1  OutDataTypeStr=Inherit: Inherit via back propagation
  TrnLeft : Sum  Inputs=+-  AccumDataTypeStr=fixdt(1,4,0)  OutDataTypeStr=fixdt(1,4,0)
  TrnRight : Sum  Inputs=+-  AccumDataTypeStr=fixdt(1,4,0)  OutDataTypeStr=fixdt(1,4,0)
  TurnLeft : Constant  Value=-1  OutDataTypeStr=fixdt(1,4,0)  SampleTime=-1
  TurnRight : Constant  OutDataTypeStr=fixdt(1,4,0)  SampleTime=-1
  count_old : Delay  DelayLength=1
  count_old1 : Delay  DelayLength=1
  count_old2 : Delay  DelayLength=1
  count_old_switch : Switch  Criteria=u2 ~= 0  OutDataTypeStr=Inherit: Inherit via back propagation
  count_old_switch1 : Switch  Criteria=u2 ~= 0  OutDataTypeStr=Inherit: Inherit via back propagation
  new_value : Delay  DelayLength=1
  nothing : Constant  Value=0  OutDataTypeStr=fixdt(1,4,0)  SampleTime=-1
  nothing1 : Constant  Value=0  OutDataTypeStr=fixdt(1,4,0)  SampleTime=-1
  speed_old_switch : Switch  Threshold=1  OutDataTypeStr=Inherit: Inherit via back propagation
  Dir : Outport
  wires:
  A/1 -> TrnLeft/2, Add/1, count_old_switch/1
  count_old_switch/1 -> count_old/1
  count_old/1 -> count_old_switch/3, Add/2
  TurnRight/1 -> T_count_switch/1
  Add/1 -> TrnRight/1, count_old_switch/2
  T_count_switch/1 -> Change/1, Add2/1
  Save_Direction/1 -> count_old2/1
  B/1 -> TrnRight/2, Add1/1, count_old_switch1/1
  count_old_switch1/1 -> count_old1/1
  count_old1/1 -> count_old_switch1/3, Add1/2
  Add1/1 -> TrnLeft/1, count_old_switch1/2
  TrnRight/1 -> Scope6/1, T_count_switch/2
  new_value/1 -> Save_Direction/1
  TrnLeft/1 -> speed_old_switch/2, Scope6/2
  TurnLeft/1 -> speed_old_switch/1
  nothing/1 -> speed_old_switch/3
  nothing1/1 -> T_count_switch/3
  speed_old_switch/1 -> Change/2, Add2/2
  Add2/1 -> Scope6/4, new_value/1
  Change/1 -> Change1/1
  Change1/1 -> Scope6/3, Save_Direction/2
  count_old2/1 -> Save_Direction/3, Dir/1

== system Encoder_Zynq/IncreEncoder_V18/Counter_speed ==
  note: 1 for one cycle if edge recognized
  note: Check if count is to small
  note: Check if count is to big
  note: Reset
  note: Count
  Enable_ctr : Inport
  Reset : Inport  Port=2
  IncsPerTurn : Inport  Port=3
  Add1 : Sum  AccumDataTypeStr=int16  OutDataTypeStr=uint16
  Constant1 : Constant  Value=0  OutDataTypeStr=uint16  SampleTime=-1
  Constant2 : Constant  OutDataTypeStr=int8  SampleTime=-1
  Constant3 : Constant  Value=0  OutDataTypeStr=int8  SampleTime=-1
  Constant4 : Constant  Value=10  OutDataTypeStr=uint16  SampleTime=-1
  Detec_edge : Sum  Inputs=+-  AccumDataTypeStr=int8  OutDataTypeStr=int8
  Relational Operator : RelationalOperator  OutDataTypeStr=boolean  RndMeth=Nearest
  Reset_flag : Sum  Inputs=+-  AccumDataTypeStr=uint8  OutDataTypeStr=uint8
  Reset_when_overflow : Sum
  Resett_switch1 : Switch  Criteria=u2 ~= 0
  Resett_switch2 : Switch  Criteria=u2 ~= 0
  reset_old{,1..3} (4 alike) : Delay  DelayLength=1
  reset_old_switch : Switch  Criteria=u2 ~= 0
  reset_old_switch1 : Switch  Criteria=u2 ~= 0
  speed_old_switch1 : Switch  Threshold=1
  count : Outport
  wires:
  Reset/1 -> Reset_flag/1, reset_old_switch/1
  reset_old_switch/1 -> reset_old/1
  reset_old/1 -> reset_old_switch/3, Reset_flag/2
  Reset_flag/1 -> reset_old_switch/2, Resett_switch2/2
  Enable_ctr/1 -> Detec_edge/1, reset_old_switch1/1
  reset_old_switch1/1 -> reset_old1/1
  reset_old1/1 -> reset_old_switch1/3, Detec_edge/2
  Detec_edge/1 -> speed_old_switch1/2, reset_old_switch1/2  "1 for one cycle if edge recognized"
  Add1/1 -> Resett_switch2/3
  reset_old2/1 -> Relational Operator/1, Add1/2, count/1
  speed_old_switch1/1 -> Add1/1
  Constant3/1 -> speed_old_switch1/3
  Constant2/1 -> speed_old_switch1/1
  Constant4/1 -> Reset_when_overflow/1
  Reset_when_overflow/1 -> reset_old3/1
  Resett_switch1/1 -> reset_old2/1
  Relational Operator/1 -> Resett_switch1/2
  Constant1/1 -> Resett_switch2/1, Resett_switch1/1
  IncsPerTurn/1 -> Reset_when_overflow/2
  Resett_switch2/1 -> Resett_switch1/3
  reset_old3/1 -> Relational Operator/2

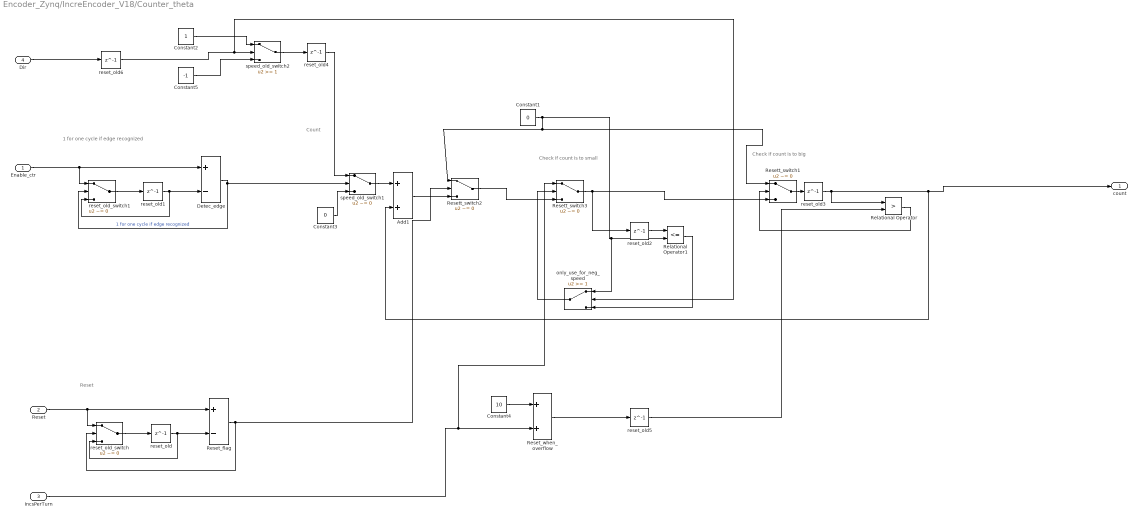
== system Encoder_Zynq/IncreEncoder_V18/Counter_theta ==
  note: 1 for one cycle if edge recognized
  note: Reset
  note: Count
  note: Check if count is to big
  note: Check if count is to small
  Enable_ctr : Inport
  Reset : Inport  Port=2
  IncsPerTurn : Inport  Port=3
  Dir : Inport  Port=4
  Add1 : Sum  AccumDataTypeStr=int16  OutDataTypeStr=int16
  Constant1 : Constant  Value=0  OutDataTypeStr=int16  SampleTime=-1
  Constant2 : Constant  OutDataTypeStr=int16  SampleTime=-1
  Constant3 : Constant  Value=0  OutDataTypeStr=int16  SampleTime=-1
  Constant4 : Constant  Value=10  OutDataTypeStr=int16  SampleTime=-1
  Constant5 : Constant  Value=-1  OutDataTypeStr=int16  SampleTime=-1
  Detec_edge : Sum  Inputs=+-  AccumDataTypeStr=int8  OutDataTypeStr=int8
  Relational Operator : RelationalOperator  Operator=>  OutDataTypeStr=boolean  RndMeth=Nearest
  Relational Operator1 : RelationalOperator  Operator=<=  OutDataTypeStr=boolean  RndMeth=Nearest
  Reset_flag : Sum  Inputs=+-  AccumDataTypeStr=uint8  OutDataTypeStr=uint8
  Reset_when_overflow : Sum  OutDataTypeStr=int16
  Resett_switch1 : Switch  Criteria=u2 ~= 0  OutDataTypeStr=int16
  Resett_switch2 : Switch  Criteria=u2 ~= 0  OutDataTypeStr=int16
  Resett_switch3 : Switch  Criteria=u2 ~= 0  OutDataTypeStr=int16
  only_use_for_neg_speed : Switch  Threshold=1
  reset_old{,1..6} (7 alike) : Delay  DelayLength=1
  reset_old_switch : Switch  Criteria=u2 ~= 0
  reset_old_switch1 : Switch  Criteria=u2 ~= 0
  speed_old_switch1 : Switch  Criteria=u2 ~= 0
  speed_old_switch2 : Switch  Threshold=1
  count : Outport
  wires:
  Reset/1 -> Reset_flag/1, reset_old_switch/1
  reset_old_switch/1 -> reset_old/1
  reset_old/1 -> reset_old_switch/3, Reset_flag/2
  Reset_flag/1 -> reset_old_switch/2, Resett_switch2/2
  Enable_ctr/1 -> Detec_edge/1, reset_old_switch1/1
  reset_old_switch1/1 -> reset_old1/1
  reset_old1/1 -> reset_old_switch1/3, Detec_edge/2
  Detec_edge/1 -> speed_old_switch1/2, reset_old_switch1/2  "1 for one cycle if edge recognized"
  Add1/1 -> Resett_switch2/3
  speed_old_switch1/1 -> Add1/1
  Constant3/1 -> speed_old_switch1/3
  Constant2/1 -> speed_old_switch2/1
  Constant4/1 -> Reset_when_overflow/1
  Reset_when_overflow/1 -> reset_old5/1
  IncsPerTurn/1 -> Resett_switch3/1, Reset_when_overflow/2
  Dir/1 -> reset_old6/1
  Constant5/1 -> speed_old_switch2/3
  speed_old_switch2/1 -> reset_old4/1
  reset_old3/1 -> Add1/2, count/1, Relational Operator/1
  Resett_switch1/1 -> reset_old3/1
  Relational Operator/1 -> Resett_switch1/2
  Constant1/1 -> Resett_switch2/1, Resett_switch1/1, only_use_for_neg_speed/1, Relational Operator1/2
  Resett_switch3/1 -> reset_old2/1, Resett_switch1/3
  Resett_switch2/1 -> Resett_switch3/3
  reset_old2/1 -> Relational Operator1/1
  Relational Operator1/1 -> only_use_for_neg_speed/3
  only_use_for_neg_speed/1 -> Resett_switch3/2
  reset_old4/1 -> speed_old_switch1/1
  reset_old5/1 -> Relational Operator/2
  reset_old6/1 -> only_use_for_neg_speed/2, speed_old_switch2/2
